simulink model "LabQues2_DCmotorControl_PresetModel_2"  (R2025a)
settings: Solver=VariableStepAuto  StartTime=0.0  StopTime=15.0  RelTol=1e-3
libraries: spsDCVoltageSourceLib x2, spsDCMachineLib x1, spsDiodeLib x1, spsGroundLib x1, spsIdealSwitchLib x1, simulink x1, sps_lib x1
settings Model: Creator=divyamgoyal  LastModifiedBy=aditl

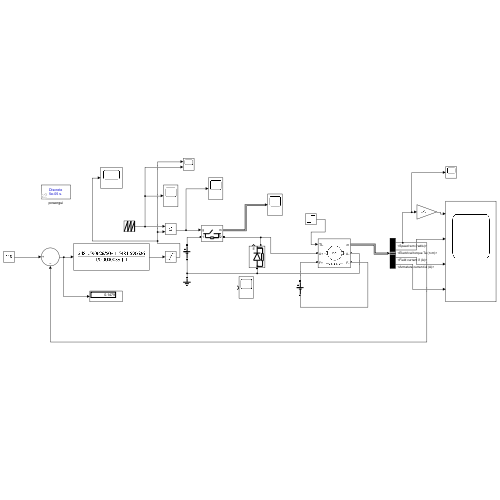
[thumbnail: Simulink's stored preview of the top-level diagram]
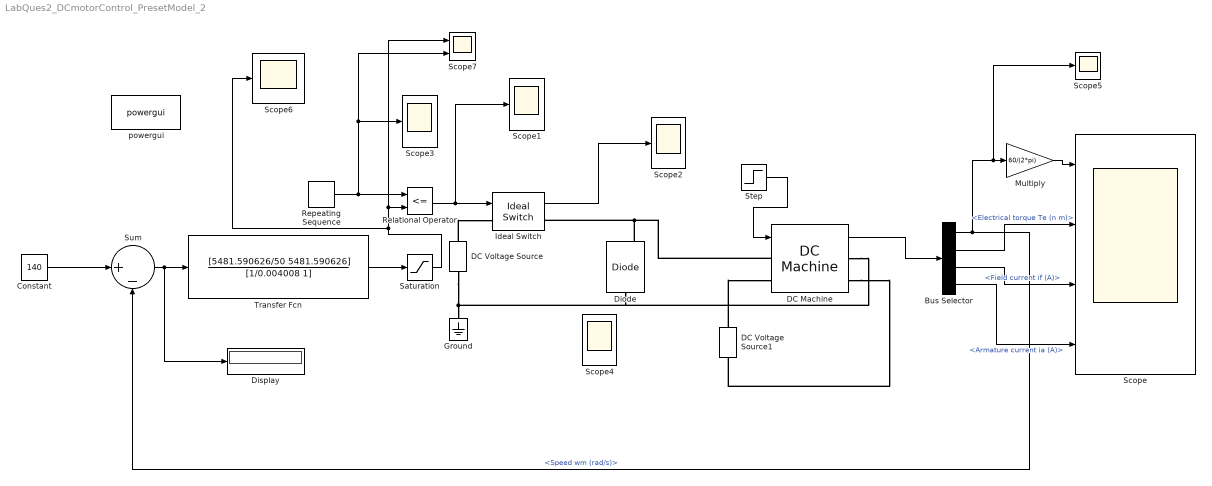
== system LabQues2_DCmotorControl_PresetModel_2 ==
  Bus Selector : BusSelector  OutputSignals=Speed wm (rad/s),Electrical torque Te (n m),Field current if (A),Armature current ia (A)
  Constant : Constant  Value=140  SampleTime=5e-5
  DC Machine : spsDCMachineLib/DC Machine  PresetModel=02: 5HP 240V 1750RPM Field:150V  MechanicalLoad=Torque TL  FieldType=Wound  ShowDetailedParameters=on  MeasurementBus=off  RLa=[0.78 0.016]  RLf=[150 112.5]  Laf=1.234  MachineConstant=Torque constant (N.m/A)  Ke=1.8  Kt=1.8  J=0.05  Bm=0.01  Tf=0  w0=0  Ifinit=1  TsPowergui=0  TsBlock=-1
  DC Voltage Source : spsDCVoltageSourceLib/DC Voltage Source  Amplitude=240  Measurements=None
  DC Voltage Source1 : spsDCVoltageSourceLib/DC Voltage Source  Amplitude=150  Measurements=None
  Diode : spsDiodeLib/Diode  Ron=0.001  Lon=0  Vf=0.8  IC=0  UseSnubber=0  Rs=500  Cs=250e-9  Measurements=on
  Display : Display
  Ground : spsGroundLib/Ground  LConnTagsString=a
  Ideal Switch : spsIdealSwitchLib/Ideal Switch  Ron=0.001  Lon=0  IC=0  Rs=1e5  Cs=inf  Measurements=on
  Multiply : Gain  Gain=60/(2*pi)
  Relational Operator : RelationalOperator  Operator=<=  OutDataTypeStr=boolean  RndMeth=Simplest  InputSameDT=off
  Repeating Sequence : simulink/Sources/Repeating Sequence  rep_seq_t=[0 0.01]  rep_seq_y=[0 100]
  Saturation : Saturate  UpperLimit=100  LowerLimit=0
  Scope : Scope  NumInputPorts=4
      settings: ActiveDisplayYMinimum=-247.75382605236194  ActiveDisplayYMaximum=2325.2765973934142
  Scope{1..6} (6 alike) : Scope
      Scope1 settings: ActiveDisplayYMinimum=-0.12499999999999997  ActiveDisplayYMaximum=1.125
      Scope2 settings: ActiveDisplayYMinimum=-25.944719994162121  ActiveDisplayYMaximum=243.502395864514  DataLoggingVariableName=ScopeData2
      Scope3 settings: ActiveDisplayYMinimum=64.034431137723843  ActiveDisplayYMaximum=72.267964071855488  DataLoggingVariableName=ScopeData3
      Scope4 settings: ActiveDisplayYMinimum=-1.0799328587514145E+9  ActiveDisplayYMaximum=9.8985672279656525E+9  DataLoggingVariableName=ScopeData4
      Scope5 settings: ActiveDisplayYMinimum=-25.810675934675746  ActiveDisplayYMaximum=242.29599932913663  DataLoggingVariableName=ScopeData5
      Scope6 settings: ActiveDisplayYMinimum=-12.499999999999996  ActiveDisplayYMaximum=112.5  DataLoggingVariableName=ScopeData6
  Scope7 : Scope  NumInputPorts=2
      settings: ActiveDisplayYMinimum=-1840.0423387634498  ActiveDisplayYMaximum=315.56025986260425  DataLoggingVariableName=ScopeData7
  Step : Step  Time=7  SampleTime=0
  Sum : Sum  Inputs=|+-
  Transfer Fcn : TransferFcn  Numerator=[5481.590626/50 5481.590626]  Denominator=[1/0.004008 1]  ParameterTunability=Unconstrained
  powergui : sps_lib/powergui  Priority=1  SimulationMode=Discrete  SampleTime=50e-6  frequency=60  Iterations=50  frequencyindice=0  Pbase=100e6  ErrMax=1e-4  UnitsV=kV  UnitsW=MW  buscounter=0  FunctionMessages=off  echomessages=off  EnableUseOfTLC=off  CurrentSourceSwitches=off  DisableSnubberDevices=off  DisableRonSwitches=off  DisableVfSwitches=off  DisplayEquations=off  AutomaticDiscreteSolvers=off  SolverType=Tustin/Backward Euler (TBE)  Interpol=off  ExternalGateDelay=off  methode=off  Ts=100  x0status=blocks  SPID=on  SwTol=0  HookPort=off  NonlinearTolerance=1e-4  nMaxIteration=100  ContinueOnMaxIteration=off  RestoreLinks=warning  ResistiveCurrentMeasurement=off  Frange=[0:2:500]  Ylog=off  Xlog=on  ShowGrid=off  save=off  variable=ZData  structure=0  ZoomFFT=off  StartTime=0.0  cycles=1  DisplayStyle=1  fundamental=60  FreqAxis=off  MaxFrequency=1000  frequencyindicesteady=1  RmsSteady=1  display=off
  wires:
  Sum/1 -> Display/1, Transfer Fcn/1
  DC Machine/1 -> Bus Selector/1
  Bus Selector/1 -> Scope5/1, Multiply/1, Sum/2  "<Speed wm (rad/s)>"
  Bus Selector/2 -> Scope/2  "<Electrical torque Te (n m)>"
  Bus Selector/3 -> Scope/3  "<Field current if (A)>"
  Bus Selector/4 -> Scope/4  "<Armature current ia (A)>"
  Repeating Sequence/1 -> Scope7/2, Scope3/1, Relational Operator/1
  Ideal Switch/1 -> Scope2/1
  Multiply/1 -> Scope/1
  Relational Operator/1 -> Scope1/1, Ideal Switch/1
  Constant/1 -> Sum/1
  Transfer Fcn/1 -> Saturation/1
  Saturation/1 -> Scope6/1, Scope7/1, Relational Operator/2
  Step/1 -> DC Machine/1
  connections:
  DC Voltage Source/RConn1 -- Ideal Switch/LConn1
  DC Voltage Source/LConn1 -- Diode/LConn1 -- DC Machine/RConn1 -- Ground/LConn1
  DC Machine/LConn1 -- Diode/RConn1 -- Ideal Switch/RConn1
  DC Voltage Source1/RConn1 -- DC Machine/LConn2
  DC Machine/RConn2 -- DC Voltage Source1/LConn1
